simulink model "mission_planner_production"  (R2015a)
settings: Solver=ode3  StartTime=0.0  StopTime=10.0  RelTol=1e-3
undefined symbols (not defined in the file): X, Y
libraries: robotlib x9
settings Model: Creator=Kelan  LastModifiedBy=Kelan
settings OptimizationCC: EnhancedBackFolding=on

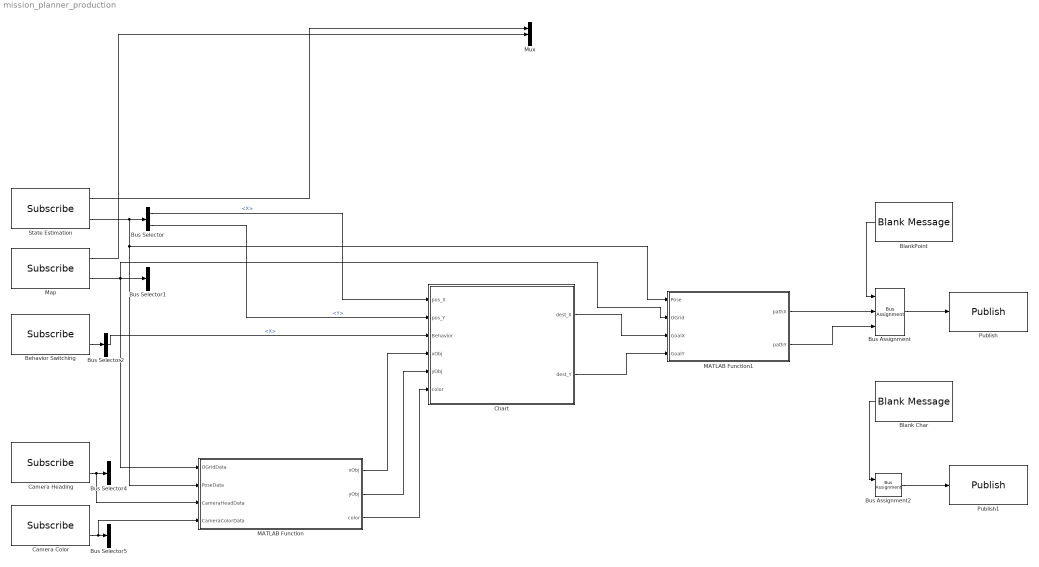
== system mission_planner_production ==
  Behavior Switching : robotlib/Subscribe  SourceLibraryInfo=This block requires Robotics System Toolbox  topicSource=Specify your own  topic=/behavior  messageType=std_msgs/UInt8  sampleTime=-1  messageQueueLength=1
  Blank Char : robotlib/Blank Message  SourceLibraryInfo=This block requires Robotics System Toolbox  messageType=std_msgs/Int16  SampleTime=inf
  BlankPoint : robotlib/Blank Message  SourceLibraryInfo=This block requires Robotics System Toolbox  messageType=geometry_msgs/Point  SampleTime=inf
  Bus Assignment : BusAssignment  AssignedSignals=X,Y
  Bus Assignment2 : BusAssignment  AssignedSignals=Data
  Bus Selector : BusSelector  OutputSignals=Pose.Position.X,Pose.Position.Y
  Bus Selector1 : BusSelector  OutputSignals=Data
  Bus Selector2 : BusSelector  OutputSignals=X
  Bus Selector4 : BusSelector  OutputSignals=X,Y,Z
  Bus Selector5 : BusSelector  OutputSignals=X,Y,Z
  Camera Color : robotlib/Subscribe  SourceLibraryInfo=This block requires Robotics System Toolbox  topicSource=Specify your own  topic=/cameraColor  messageType=std_msgs/UInt8  sampleTime=-1  messageQueueLength=1
  Camera Heading : robotlib/Subscribe  SourceLibraryInfo=This block requires Robotics System Toolbox  topicSource=Specify your own  topic=/cameraHead  messageType=geometry_msgs/Pose  sampleTime=-1  messageQueueLength=1
  Chart : Stateflow chart  TreatAsAtomicUnit=on
  MATLAB Function : MATLAB Function  TreatAsAtomicUnit=on
  MATLAB Function1 : MATLAB Function  TreatAsAtomicUnit=on
  Map : robotlib/Subscribe  SourceLibraryInfo=This block requires Robotics System Toolbox  topicSource=Specify your own  topic=/map  messageType=nav_msgs/OccupancyGrid  sampleTime=-1  messageQueueLength=1
  Mux : Mux  Inputs=3
  Publish : robotlib/Publish  SourceLibraryInfo=This block requires Robotics System Toolbox  topicSource=Specify your own  topic=/GoTo  messageType=geometry_msgs/Point  messageQueueLength=1
  Publish1 : robotlib/Publish  SourceLibraryInfo=This block requires Robotics System Toolbox  topicSource=Specify your own  topic=/maneuver_command  messageType=std_msgs/Int16  messageQueueLength=1
  State Estimation : robotlib/Subscribe  SourceLibraryInfo=This block requires Robotics System Toolbox  topicSource=Specify your own  topic=/slam_pose_out  messageType=geometry_msgs/PoseStamped  sampleTime=-1  messageQueueLength=1
  wires:
  BlankPoint/1 -> Bus Assignment/1
  Bus Assignment/1 -> Publish/1
  State Estimation/2 -> MATLAB Function1/1(Pose), MATLAB Function/2(PoseData), Bus Selector/1
  Map/2 -> MATLAB Function1/2(OGrid), MATLAB Function/1(OGridData), Bus Selector1/1
  Blank Char/1 -> Bus Assignment2/1
  Bus Assignment2/1 -> Publish1/1
  State Estimation/1 -> Mux/1
  Map/1 -> Mux/2
  Bus Selector/1 -> Chart/1(pos_X)  "<X>"
  Bus Selector/2 -> Chart/2(pos_Y)  "<Y>"
  Camera Heading/2 -> MATLAB Function/3(CameraHeadData), Bus Selector4/1
  Camera Color/2 -> MATLAB Function/4(CameraColorData), Bus Selector5/1
  MATLAB Function1/1(pathX) -> Bus Assignment/2
  MATLAB Function1/2(pathY) -> Bus Assignment/3
  Chart/2(dest_Y) -> MATLAB Function1/4(GoalY)
  Chart/1(dest_X) -> MATLAB Function1/3(GoalX)
  Behavior Switching/2 -> Bus Selector2/1
  Bus Selector2/1 -> Chart/3(Behavior)  "<X>"
  MATLAB Function/3(color) -> Chart/6(color)
  MATLAB Function/1(xObj) -> Chart/4(xObj)
  MATLAB Function/2(yObj) -> Chart/5(yObj)

== matlab function mission_planner_production/MATLAB Function1 ==
  data: Pose input; OGrid input; GoalX input; GoalY input; pathX output; pathY output
function [pathX, pathY] = fcn(Pose, OGrid, GoalX, GoalY)
%#codegen

% Interpret data
    currX = roundn(PoseData.Pose.Pose.Position.X, -1);
    currY = roundn(PoseData.Pose.Pose.Position.Y, -1);
    currPos = [currX, currY];


% Create a D* Object using the map
    [map, currPos] = convO2M(OGrid, currPos)
    goal = [GoalX, GoalY];
    start= currPos;
    MapConversionFinished=1
    ds = Dstar(map);
    DSMapFinished=1
    ds.plan(goal);

    spath = ds.path(start);

    spath


    % Publish path information
    pathX = spath(:, 1);
    pathY = spath(:, 2);
end

== matlab function mission_planner_production/MATLAB Function ==
  data: OGridData input; xObj output; PoseData input; CameraHeadData input; CameraColorData input; yObj output; color output
function [xObj, yObj, color] = event_search(OGridData, PoseData, CameraHeadData, CameraColorData)
%This function returns the point of an object as xObj and yObj given angle, from LiDAR and Camera, and color, from Camera. If
%it = 6969, then it did not successfully find an object. This code currently only checks along one ray. Still need to add code to check the entire area of possibility.

% Interpret data
currentX = roundn(PoseData.Pose.Pose.Position.X, -1);   % Extracts current location in OGrid
currentY = roundn(PoseData.Pose.Pose.Position.Y, -1);   % and rounds to nearest tenth
rotZ = PoseData.Pose.Pose.Orientation.Z;                % Angle relative to start, 0. from -1-0-1
phi = CameraHeadData;                                   % Angle of object from center, DEGREES
convFLG = 0
map = readBinaryOccupancyGrid(OGridData);               % Conv. prob. OGrid to Bin. OGrid
convFLG = 1
if rotZ>0
     theta = rotZ*180;                                  % theta is angle relative to start=0*
else if rotZ<0                                          % in degrees
        theta = 360+rotZ*180;
    else
        theta=0;
    end
end

objAngle = theta-phi;
if objAngle>360
     objAngle-360;
end
angleError = 7;                                         % Guessed angle error, +/-


% We now have the x and y location in ogrid, the ogrid, the current
% heading, the current angle of object, and object color.

% Extract objective position data
xRay = currentX;
yRay = currentY;
xEst = currentX;
yEst = currentY;
angle = objAngle;
xObj = 6969;
yObj = 6969;
occupied = 0;
camera = CameraColorData;
    for dist = 1:50                             % Only checks up to 5m away
        
        xRay = xRay + 0.1 * cosd(angle);
        yRay = yRay + 0.1 * sind(angle);
        xEst = roundn(xRay, -1);                % The next point in the OGrid along ray
        yEst = roundn(yRay, -1);

        occupied = getOccupancy(map, [xEst, yEst]);
        if occupied                             % If occupied, return and break loop.
            xObj = xEst;
            yObj = yEst;
            break
        end
    end
    if occupied                                 % breaks while loop if condition is met
        break
    end
    % TODO: Add error increments, possibly use Nathan's code to get all
    % points in the cone of possible objects.
end

== stateflow chart mission_planner_production/Chart ==
  state steady_state
    entry:
  state Preliminary Task
    (default) -> (junction 54) : % Entry Buoy
    (junction 54) -> (junction 57) [order 1] : [color == 1]
    (junction 54) -> (junction 56) [order 2]
    (junction 57) -> (junction 58) : {destX = posX + 50;}
    (junction 56) -> (junction 59) [order 1] : [color == 2]
    (junction 56) -> (junction 55) [order 2]
    (junction 59) -> (junction 60) : {destY = posY+50;}
    (junction 60) -> (junction 55)
    (junction 58) -> (junction 60)
    (junction 55) -> (junction 76) : % End Search
    (junction 76) -> (junction 73)
    (junction 73) -> (junction 75) [order 1] : [color = 0]
    (junction 75) -> (junction 72) : {destX = posX + 50;}
    (junction 72) -> (junction 73)
    (junction 73) -> (junction 83) [order 2] : % End Buoy
    (junction 83) -> (junction 86) [order 1] : [color == 1]
    (junction 83) -> (junction 85) [order 2]
    (junction 86) -> (junction 87) : {destX = posX + 10;}
    (junction 85) -> (junction 88) [order 1] : [color == 2]
    (junction 85) -> (junction 84) [order 2]
    (junction 88) -> (junction 89) : {destY = posY + 10;}
    (junction 89) -> (junction 84)
    (junction 87) -> (junction 89)
    (junction 84) -> (junction 101) : % End Condition
    (junction 101) -> (junction 104) [order 1] : [posX > xObj]
    (junction 101) -> (junction 103) [order 2]
    (junction 104) -> (junction 105) : {destX = posX;}
    (junction 103) -> (junction 106) [order 1] : [posY > yObj]
    (junction 103) -> (junction 102) [order 2]
    (junction 106) -> (junction 107) : {destY = posY;}
    (junction 107) -> (junction 102)
    (junction 105) -> (junction 107)
    (junction 102) -> (junction 108)
  state Survey [group]
    (junction 8) -> (junction 10) : {loop=0}
    (junction 10) -> (junction 9) [order 1] : [detected=0]
    (junction 9) -> (junction 11) : {dest_Y = pos_Y+10;}
    (junction 12) -> (junction 10) [order 1] : {loop=loop+1}
    (default) -> (junction 10)
    (junction 10) -> (junction 18) [order 2]
    (junction 11) -> (junction 12) : {index=0;}
    (junction 12) -> (junction 13) [order 2] : [(detected=0)&&(index<12)]
    (junction 17) -> (junction 12) : {index=index+1;}
    (junction 13) -> (junction 14) [order 1] : [loop%2=0]
    (junction 13) -> (junction 15) [order 2] : {dest_X = pos_X - 10;}
    (junction 14) -> (junction 16) : {dest_X = pos_X + 10;}
    (junction 16) -> (junction 15)
    (junction 15) -> (junction 17)
    (junction 18) -> ? : [Behavior=0]
  (default) -> steady_state
  Preliminary Task -> steady_state : [Behavior=0]
  steady_state -> Preliminary Task : [Behavior ==1]
  data: dest_X output; dest_Y output; pos_X input; pos_Y input; Behavior input; xObj input; yObj input; color input
